simulink library "acc"  (R2021b)
settings: Solver=VariableStepAuto  StartTime=0.0  StopTime=10.0  RelTol=1e-3
undefined symbols (not defined in the file or in its folder): AACC_EHPSSpdCtrlMode_X_enum, AACC_EHPSSpdCtrlMode_Y_rad, ENUM__SASCALED_CALED, ENUM_BRAKEPEDAL_RELEASED, ENUM_CACENABLESTS_RUN, ENUM_DCDCENABLESTS_RUN, ENUM_EHPSCTRLMODE_FULLPWR, ENUM_EHPSCTRLMODE_NORMAL, ENUM_EHPSCTRLMODE_STEP1, ENUM_EHPSCTRLMODE_ZERO, ENUM_EHPSENABLESTS_INITIAL, ENUM_EHPSENABLESTS_READY, ENUM_EHPSENABLESTS_RUN, ENUM_PMMMODE_DRIVE, ENUM_PMMMODE_POWERUP, ENUM_TARGETGEAR_NEUTRAL, FALSE, KACC_AirPressInvalid_kpa, KACC_CACEnableFailTime_s, KACC_CACOverrunRcvTime_s, KACC_CACOverrunTime_min, KACC_CACOverTempDelayTime_s, KACC_CACOverTempRcv_s, KACC_CACPresLow_kPa, KACC_CACPressureSWRev_flg, KACC_CACPresWarn_kPa, KACC_CACPresWarn_ovrdflg_flg, KACC_CACPresWarn_ovrdval_flg, KACC_CACStopTime_s, KACC_CACTemp_C, KACC_CACTempRev_C, KACC_CACTempStop_C, KACC_CACTempWarn_C, KACC_CACValid_flg, KACC_CP2VAutoTracH_enum, KACC_CP2VDamStiffReqFA_pct, KACC_CP2VDamStiffReqLA_pct, KACC_CP2VDamStiffReqRA_pct, KACC_CP2VKneeCtrlMReq_enum, KACC_CP2VKneeReqFA_enum, KACC_CP2VKneeReqRA_enum, KACC_CP2VKneeReqRSide_enum, KACC_CP2VLA1PosCmd_enum, KACC_CP2VLA2PosCmd_enum, KACC_CP2VLvCtrlModeReq_enum, KACC_CP2VNLvReqFA_enum, KACC_CP2VNLvReqRA_enum, KACC_DCDCErrLvHoldtime_s, KACC_DTCACCReset_flg, KACC_DTCCACOverrun_cnt, KACC_EACErrLvHoldtime_s, KACC_ECASKneeSideSW_flg, KACC_EcasSw1Down_flg, KACC_EcasSw1Up_flg, KACC_EcasSw2M2_flg, KACC_EcasSw2Stop_flg, KACC_EcasSw3Knee_flg, KACC_EcasSw3M1_flg, KACC_EcasSwDebounceTime_s, KACC_ECASSwitch_flg ... (+30)
libraries: hcu_lib x20, simulink x3
(part 2 of 3)

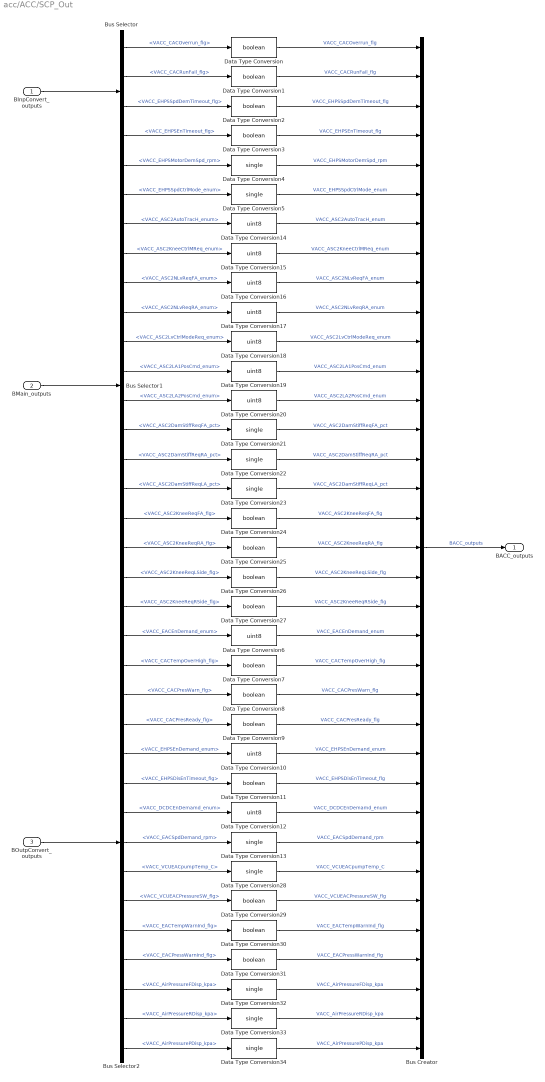
== system acc/ACC/SCP_Out ==
  BInpConvert_outputs : Inport
  BMain_outputs : Inport  Port=2
  BOutpConvert_outputs : Inport  Port=3
  Bus Creator : BusCreator  Inputs=35  OutDataTypeStr=Bus:BACC_outputs  NonVirtualBus=on
  Bus Selector : BusSelector  OutputSignals=VACC_CACOverrun_flg,VACC_CACRunFail_flg,VACC_EHPSSpdDemTimeout_flg,VACC_EHPSEnTimeout_flg
  Bus Selector1 : BusSelector  OutputSignals=VACC_EHPSMotorDemSpd_rpm,VACC_EHPSSpdCtrlMode_enum,VACC_ASC2AutoTracH_enum,VACC_ASC2KneeCtrlMReq_enum,VACC_ASC2NLvReqFA_enum,VACC_ASC2NLvReqRA_enum,VACC_ASC2LvCtrlModeReq_enum,VACC_ASC2LA1PosCmd_enum,VACC_ASC2LA2PosCmd_enum,VACC_ASC2DamStiffReqFA_pct,VACC_ASC2DamStiffReqRA_pct,VACC_ASC2DamStiffReqLA_pct,VACC_ASC2KneeReqFA_flg,VACC_ASC2KneeReqRA_flg,VACC_ASC2KneeReqLSide_flg,VACC_ASC2KneeReqRSide_flg
  Bus Selector2 : BusSelector  OutputSignals=VACC_EACEnDemand_enum,VACC_CACTempOverHigh_flg,VACC_CACPresWarn_flg,VACC_CACPresReady_flg,VACC_EHPSEnDemand_enum,VACC_EHPSDisEnTimeout_flg,VACC_DCDCEnDemamd_enum,VACC_EACSpdDemand_rpm,VACC_VCUEACpumpTemp_C,VACC_VCUEACPressureSW_flg,VACC_EACTempWarnInd_flg,VACC_EACPressWarnInd_flg,VACC_AirPressureFDisp_kpa,VACC_AirPressureRDisp_kpa,VACC_AirPressurePDisp_kpa
  Data Type Conversion{,1..3,7..9,11,24..27,29..31} (15 alike) : DataTypeConversion  OutDataTypeStr=boolean
  Data Type Conversion{6,10,12,14..20} (10 alike) : DataTypeConversion  OutDataTypeStr=uint8
  Data Type Conversion{4..5,13,21..23,28,32..34} (10 alike) : DataTypeConversion  OutDataTypeStr=single
  BACC_outputs : Outport
  wires:
  BInpConvert_outputs/1 -> Bus Selector/1
  BMain_outputs/1 -> Bus Selector1/1
  BOutpConvert_outputs/1 -> Bus Selector2/1
  Bus Selector/1 -> Data Type Conversion/1  "<VACC_CACOverrun_flg>"
  Bus Selector/2 -> Data Type Conversion1/1  "<VACC_CACRunFail_flg>"
  Bus Selector/3 -> Data Type Conversion2/1  "<VACC_EHPSSpdDemTimeout_flg>"
  Bus Selector/4 -> Data Type Conversion3/1  "<VACC_EHPSEnTimeout_flg>"
  Bus Selector1/1 -> Data Type Conversion4/1  "<VACC_EHPSMotorDemSpd_rpm>"
  Bus Selector1/2 -> Data Type Conversion5/1  "<VACC_EHPSSpdCtrlMode_enum>"
  Bus Selector2/1 -> Data Type Conversion6/1  "<VACC_EACEnDemand_enum>"
  Bus Selector2/2 -> Data Type Conversion7/1  "<VACC_CACTempOverHigh_flg>"
  Bus Selector2/3 -> Data Type Conversion8/1  "<VACC_CACPresWarn_flg>"
  Bus Selector2/4 -> Data Type Conversion9/1  "<VACC_CACPresReady_flg>"
  Bus Selector2/5 -> Data Type Conversion10/1  "<VACC_EHPSEnDemand_enum>"
  Bus Selector2/6 -> Data Type Conversion11/1  "<VACC_EHPSDisEnTimeout_flg>"
  Bus Selector2/7 -> Data Type Conversion12/1  "<VACC_DCDCEnDemamd_enum>"
  Bus Selector2/8 -> Data Type Conversion13/1  "<VACC_EACSpdDemand_rpm>"
  Data Type Conversion/1 -> Bus Creator/1  "VACC_CACOverrun_flg"
  Data Type Conversion1/1 -> Bus Creator/2  "VACC_CACRunFail_flg"
  Data Type Conversion2/1 -> Bus Creator/3  "VACC_EHPSSpdDemTimeout_flg"
  Data Type Conversion3/1 -> Bus Creator/4  "VACC_EHPSEnTimeout_flg"
  Data Type Conversion4/1 -> Bus Creator/5  "VACC_EHPSMotorDemSpd_rpm"
  Data Type Conversion5/1 -> Bus Creator/6  "VACC_EHPSSpdCtrlMode_enum"
  Bus Creator/1 -> BACC_outputs/1  "BACC_outputs"
  Bus Selector1/3 -> Data Type Conversion14/1  "<VACC_ASC2AutoTracH_enum>"
  Bus Selector1/4 -> Data Type Conversion15/1  "<VACC_ASC2KneeCtrlMReq_enum>"
  Bus Selector1/5 -> Data Type Conversion16/1  "<VACC_ASC2NLvReqFA_enum>"
  Bus Selector1/6 -> Data Type Conversion17/1  "<VACC_ASC2NLvReqRA_enum>"
  Bus Selector1/7 -> Data Type Conversion18/1  "<VACC_ASC2LvCtrlModeReq_enum>"
  Bus Selector1/8 -> Data Type Conversion19/1  "<VACC_ASC2LA1PosCmd_enum>"
  Bus Selector1/9 -> Data Type Conversion20/1  "<VACC_ASC2LA2PosCmd_enum>"
  Bus Selector1/10 -> Data Type Conversion21/1  "<VACC_ASC2DamStiffReqFA_pct>"
  Bus Selector1/11 -> Data Type Conversion22/1  "<VACC_ASC2DamStiffReqRA_pct>"
  Bus Selector1/12 -> Data Type Conversion23/1  "<VACC_ASC2DamStiffReqLA_pct>"
  Bus Selector1/13 -> Data Type Conversion24/1  "<VACC_ASC2KneeReqFA_flg>"
  Bus Selector1/14 -> Data Type Conversion25/1  "<VACC_ASC2KneeReqRA_flg>"
  Bus Selector1/15 -> Data Type Conversion26/1  "<VACC_ASC2KneeReqLSide_flg>"
  Bus Selector1/16 -> Data Type Conversion27/1  "<VACC_ASC2KneeReqRSide_flg>"
  Bus Selector2/9 -> Data Type Conversion28/1  "<VACC_VCUEACpumpTemp_C>"
  Bus Selector2/10 -> Data Type Conversion29/1  "<VACC_VCUEACPressureSW_flg>"
  Bus Selector2/11 -> Data Type Conversion30/1  "<VACC_EACTempWarnInd_flg>"
  Bus Selector2/12 -> Data Type Conversion31/1  "<VACC_EACPressWarnInd_flg>"
  Bus Selector2/13 -> Data Type Conversion32/1  "<VACC_AirPressureFDisp_kpa>"
  Bus Selector2/14 -> Data Type Conversion33/1  "<VACC_AirPressureRDisp_kpa>"
  Bus Selector2/15 -> Data Type Conversion34/1  "<VACC_AirPressurePDisp_kpa>"
  Data Type Conversion14/1 -> Bus Creator/7  "VACC_ASC2AutoTracH_enum"
  Data Type Conversion15/1 -> Bus Creator/8  "VACC_ASC2KneeCtrlMReq_enum"
  Data Type Conversion16/1 -> Bus Creator/9  "VACC_ASC2NLvReqFA_enum"
  Data Type Conversion17/1 -> Bus Creator/10  "VACC_ASC2NLvReqRA_enum"
  Data Type Conversion18/1 -> Bus Creator/11  "VACC_ASC2LvCtrlModeReq_enum"
  Data Type Conversion19/1 -> Bus Creator/12  "VACC_ASC2LA1PosCmd_enum"
  Data Type Conversion20/1 -> Bus Creator/13  "VACC_ASC2LA2PosCmd_enum"
  Data Type Conversion21/1 -> Bus Creator/14  "VACC_ASC2DamStiffReqFA_pct"
  Data Type Conversion22/1 -> Bus Creator/15  "VACC_ASC2DamStiffReqRA_pct"
  Data Type Conversion23/1 -> Bus Creator/16  "VACC_ASC2DamStiffReqLA_pct"
  Data Type Conversion24/1 -> Bus Creator/17  "VACC_ASC2KneeReqFA_flg"
  Data Type Conversion25/1 -> Bus Creator/18  "VACC_ASC2KneeReqRA_flg"
  Data Type Conversion26/1 -> Bus Creator/19  "VACC_ASC2KneeReqLSide_flg"
  Data Type Conversion27/1 -> Bus Creator/20  "VACC_ASC2KneeReqRSide_flg"
  Data Type Conversion6/1 -> Bus Creator/21  "VACC_EACEnDemand_enum"
  Data Type Conversion7/1 -> Bus Creator/22  "VACC_CACTempOverHigh_flg"
  Data Type Conversion8/1 -> Bus Creator/23  "VACC_CACPresWarn_flg"
  Data Type Conversion9/1 -> Bus Creator/24  "VACC_CACPresReady_flg"
  Data Type Conversion10/1 -> Bus Creator/25  "VACC_EHPSEnDemand_enum"
  Data Type Conversion11/1 -> Bus Creator/26  "VACC_EHPSDisEnTimeout_flg"
  Data Type Conversion12/1 -> Bus Creator/27  "VACC_DCDCEnDemamd_enum"
  Data Type Conversion13/1 -> Bus Creator/28  "VACC_EACSpdDemand_rpm"
  Data Type Conversion28/1 -> Bus Creator/29  "VACC_VCUEACpumpTemp_C"
  Data Type Conversion29/1 -> Bus Creator/30  "VACC_VCUEACPressureSW_flg"
  Data Type Conversion30/1 -> Bus Creator/31  "VACC_EACTempWarnInd_flg"
  Data Type Conversion31/1 -> Bus Creator/32  "VACC_EACPressWarnInd_flg"
  Data Type Conversion32/1 -> Bus Creator/33  "VACC_AirPressureFDisp_kpa"
  Data Type Conversion33/1 -> Bus Creator/34  "VACC_AirPressureRDisp_kpa"
  Data Type Conversion34/1 -> Bus Creator/35  "VACC_AirPressurePDisp_kpa"

== system acc/ACC/Input_Convert/ EcasSw1Down Debounce ==
  signal_raw : Inport
  time_limit : Inport  Port=2
  time_step : Inport  Port=3
  Add : Sum
  Add1 : Sum
  Constant : Constant  Value=FALSE
  Constant1 : Constant  Value=0
  Relational Operator : RelationalOperator  OutDataTypeStr=boolean  RndMeth=Simplest
  Switch : Switch  Criteria=u2 ~= 0
      settings: AttributesFormatString=%<Criteria>
  Switch1 : Switch  Criteria=u2 ~= 0
      settings: AttributesFormatString=%<Criteria>
  Unit Delay : UnitDelay  SampleTime=-1  HasFrameUpgradeWarning=on
  signal_out : Outport
  wires:
  signal_raw/1 -> Switch1/2, Switch/2
  Constant/1 -> Switch/3
  time_step/1 -> Add1/2, Add/1
  Unit Delay/1 -> Add/2
  Relational Operator/1 -> Switch/1
  Switch1/1 -> Unit Delay/1, Relational Operator/1
  Add/1 -> Switch1/1
  Constant1/1 -> Switch1/3
  Switch/1 -> signal_out/1
  time_limit/1 -> Add1/1
  Add1/1 -> Relational Operator/2

== system acc/ACC/Input_Convert/ EcasSw1Up Debounce ==
  signal_raw : Inport
  time_limit : Inport  Port=2
  time_step : Inport  Port=3
  Add : Sum
  Add1 : Sum
  Constant : Constant  Value=FALSE
  Constant1 : Constant  Value=0
  Relational Operator : RelationalOperator  OutDataTypeStr=boolean  RndMeth=Simplest
  Switch : Switch  Criteria=u2 ~= 0
      settings: AttributesFormatString=%<Criteria>
  Switch1 : Switch  Criteria=u2 ~= 0
      settings: AttributesFormatString=%<Criteria>
  Unit Delay : UnitDelay  SampleTime=-1  HasFrameUpgradeWarning=on
  signal_out : Outport
  wires:
  signal_raw/1 -> Switch1/2, Switch/2
  Constant/1 -> Switch/3
  time_step/1 -> Add1/2, Add/1
  Unit Delay/1 -> Add/2
  Relational Operator/1 -> Switch/1
  Switch1/1 -> Unit Delay/1, Relational Operator/1
  Add/1 -> Switch1/1
  Constant1/1 -> Switch1/3
  Switch/1 -> signal_out/1
  time_limit/1 -> Add1/1
  Add1/1 -> Relational Operator/2

== system acc/ACC/Input_Convert/ EcasSw2Stop Debounce ==
  signal_raw : Inport
  time_limit : Inport  Port=2
  time_step : Inport  Port=3
  Add : Sum
  Add1 : Sum
  Constant : Constant  Value=FALSE
  Constant1 : Constant  Value=0
  Relational Operator : RelationalOperator  OutDataTypeStr=boolean  RndMeth=Simplest
  Switch : Switch  Criteria=u2 ~= 0
      settings: AttributesFormatString=%<Criteria>
  Switch1 : Switch  Criteria=u2 ~= 0
      settings: AttributesFormatString=%<Criteria>
  Unit Delay : UnitDelay  SampleTime=-1  HasFrameUpgradeWarning=on
  signal_out : Outport
  wires:
  signal_raw/1 -> Switch1/2, Switch/2
  Constant/1 -> Switch/3
  time_step/1 -> Add1/2, Add/1
  Unit Delay/1 -> Add/2
  Relational Operator/1 -> Switch/1
  Switch1/1 -> Unit Delay/1, Relational Operator/1
  Add/1 -> Switch1/1
  Constant1/1 -> Switch1/3
  Switch/1 -> signal_out/1
  time_limit/1 -> Add1/1
  Add1/1 -> Relational Operator/2

== system acc/ACC/Input_Convert/EcasSw2M2 Debounce ==
  signal_raw : Inport
  time_limit : Inport  Port=2
  time_step : Inport  Port=3
  Add : Sum
  Add1 : Sum
  Constant : Constant  Value=FALSE
  Constant1 : Constant  Value=0
  Relational Operator : RelationalOperator  OutDataTypeStr=boolean  RndMeth=Simplest
  Switch : Switch  Criteria=u2 ~= 0
      settings: AttributesFormatString=%<Criteria>
  Switch1 : Switch  Criteria=u2 ~= 0
      settings: AttributesFormatString=%<Criteria>
  Unit Delay : UnitDelay  SampleTime=-1  HasFrameUpgradeWarning=on
  signal_out : Outport
  wires:
  signal_raw/1 -> Switch1/2, Switch/2
  Constant/1 -> Switch/3
  time_step/1 -> Add1/2, Add/1
  Unit Delay/1 -> Add/2
  Relational Operator/1 -> Switch/1
  Switch1/1 -> Unit Delay/1, Relational Operator/1
  Add/1 -> Switch1/1
  Constant1/1 -> Switch1/3
  Switch/1 -> signal_out/1
  time_limit/1 -> Add1/1
  Add1/1 -> Relational Operator/2

== system acc/ACC/Input_Convert/EcasSw3Knee Debounce ==
  signal_raw : Inport
  time_limit : Inport  Port=2
  time_step : Inport  Port=3
  Add : Sum
  Add1 : Sum
  Constant : Constant  Value=FALSE
  Constant1 : Constant  Value=0
  Relational Operator : RelationalOperator  OutDataTypeStr=boolean  RndMeth=Simplest
  Switch : Switch  Criteria=u2 ~= 0
      settings: AttributesFormatString=%<Criteria>
  Switch1 : Switch  Criteria=u2 ~= 0
      settings: AttributesFormatString=%<Criteria>
  Unit Delay : UnitDelay  SampleTime=-1  HasFrameUpgradeWarning=on
  signal_out : Outport
  wires:
  signal_raw/1 -> Switch1/2, Switch/2
  Constant/1 -> Switch/3
  time_step/1 -> Add1/2, Add/1
  Unit Delay/1 -> Add/2
  Relational Operator/1 -> Switch/1
  Switch1/1 -> Unit Delay/1, Relational Operator/1
  Add/1 -> Switch1/1
  Constant1/1 -> Switch1/3
  Switch/1 -> signal_out/1
  time_limit/1 -> Add1/1
  Add1/1 -> Relational Operator/2

== system acc/ACC/Input_Convert/EcasSw3M1 Debounce ==
  signal_raw : Inport
  time_limit : Inport  Port=2
  time_step : Inport  Port=3
  Add : Sum
  Add1 : Sum
  Constant : Constant  Value=FALSE
  Constant1 : Constant  Value=0
  Relational Operator : RelationalOperator  OutDataTypeStr=boolean  RndMeth=Simplest
  Switch : Switch  Criteria=u2 ~= 0
      settings: AttributesFormatString=%<Criteria>
  Switch1 : Switch  Criteria=u2 ~= 0
      settings: AttributesFormatString=%<Criteria>
  Unit Delay : UnitDelay  SampleTime=-1  HasFrameUpgradeWarning=on
  signal_out : Outport
  wires:
  signal_raw/1 -> Switch1/2, Switch/2
  Constant/1 -> Switch/3
  time_step/1 -> Add1/2, Add/1
  Unit Delay/1 -> Add/2
  Relational Operator/1 -> Switch/1
  Switch1/1 -> Unit Delay/1, Relational Operator/1
  Add/1 -> Switch1/1
  Constant1/1 -> Switch1/3
  Switch/1 -> signal_out/1
  time_limit/1 -> Add1/1
  Add1/1 -> Relational Operator/2

== system acc/ACC/Input_Convert/Switch hold ==
  signal_in : Inport
  hold_time : Inport  Port=2
  time_step : Inport  Port=3
  Add : Sum
  Constant1 : Constant  Value=0
  Constant3 : Constant  Value=0
  Constant4 : Constant
  Detect Increase : simulink/Logic and Bit Operations/Detect Increase  vinit=0.0  OutDataTypeStr=boolean
  Relational Operator : RelationalOperator  OutDataTypeStr=boolean  RndMeth=Simplest
  Switch1 : Switch  Criteria=u2 ~= 0
      settings: AttributesFormatString=%<Criteria>
  Switch2 : Switch  Criteria=u2 ~= 0
      settings: AttributesFormatString=%<Criteria>
  Switch3 : Switch  Criteria=u2 ~= 0
      settings: AttributesFormatString=%<Criteria>
  Unit Delay : UnitDelay  SampleTime=-1  HasFrameUpgradeWarning=on
  Unit Delay1 : UnitDelay  SampleTime=-1  HasFrameUpgradeWarning=on
  signal_out : Outport
  wires:
  signal_in/1 -> Detect Increase/1
  Detect Increase/1 -> Switch1/2
  Unit Delay/1 -> Switch1/3
  Switch2/1 -> signal_out/1, Unit Delay/1
  Relational Operator/1 -> Switch2/2
  hold_time/1 -> Relational Operator/2
  Switch1/1 -> Switch3/2, Switch2/3
  Switch3/1 -> Unit Delay1/1, Relational Operator/1
  Unit Delay1/1 -> Add/2
  time_step/1 -> Add/1
  Add/1 -> Switch3/1
  Constant1/1 -> Switch3/3
  Constant3/1 -> Switch2/1
  Constant4/1 -> Switch1/1

== system acc/ACC/Input_Convert/Switch hold1 ==
  signal_in : Inport
  hold_time : Inport  Port=2
  time_step : Inport  Port=3
  Add : Sum
  Constant1 : Constant  Value=0
  Constant3 : Constant  Value=0
  Constant4 : Constant
  Detect Increase : simulink/Logic and Bit Operations/Detect Increase  vinit=0.0  OutDataTypeStr=boolean
  Relational Operator : RelationalOperator  OutDataTypeStr=boolean  RndMeth=Simplest
  Switch1 : Switch  Criteria=u2 ~= 0
      settings: AttributesFormatString=%<Criteria>
  Switch2 : Switch  Criteria=u2 ~= 0
      settings: AttributesFormatString=%<Criteria>
  Switch3 : Switch  Criteria=u2 ~= 0
      settings: AttributesFormatString=%<Criteria>
  Unit Delay : UnitDelay  SampleTime=-1  HasFrameUpgradeWarning=on
  Unit Delay1 : UnitDelay  SampleTime=-1  HasFrameUpgradeWarning=on
  signal_out : Outport
  wires:
  signal_in/1 -> Detect Increase/1
  Detect Increase/1 -> Switch1/2
  Unit Delay/1 -> Switch1/3
  Switch2/1 -> signal_out/1, Unit Delay/1
  Relational Operator/1 -> Switch2/2
  hold_time/1 -> Relational Operator/2
  Switch1/1 -> Switch3/2, Switch2/3
  Switch3/1 -> Unit Delay1/1, Relational Operator/1
  Unit Delay1/1 -> Add/2
  time_step/1 -> Add/1
  Add/1 -> Switch3/1
  Constant1/1 -> Switch3/3
  Constant3/1 -> Switch2/1
  Constant4/1 -> Switch1/1

== system acc/ACC/Input_Convert/Switch hold3 ==
  signal_in : Inport
  hold_time : Inport  Port=2
  time_step : Inport  Port=3
  Add : Sum
  Constant1 : Constant  Value=0
  Constant3 : Constant  Value=0
  Constant4 : Constant
  Detect Increase : simulink/Logic and Bit Operations/Detect Increase  vinit=0.0  OutDataTypeStr=boolean
  Relational Operator : RelationalOperator  OutDataTypeStr=boolean  RndMeth=Simplest
  Switch1 : Switch  Criteria=u2 ~= 0
      settings: AttributesFormatString=%<Criteria>
  Switch2 : Switch  Criteria=u2 ~= 0
      settings: AttributesFormatString=%<Criteria>
  Switch3 : Switch  Criteria=u2 ~= 0
      settings: AttributesFormatString=%<Criteria>
  Unit Delay : UnitDelay  SampleTime=-1  HasFrameUpgradeWarning=on
  Unit Delay1 : UnitDelay  SampleTime=-1  HasFrameUpgradeWarning=on
  signal_out : Outport
  wires:
  signal_in/1 -> Detect Increase/1
  Detect Increase/1 -> Switch1/2
  Unit Delay/1 -> Switch1/3
  Switch2/1 -> signal_out/1, Unit Delay/1
  Relational Operator/1 -> Switch2/2
  hold_time/1 -> Relational Operator/2
  Switch1/1 -> Switch3/2, Switch2/3
  Switch3/1 -> Unit Delay1/1, Relational Operator/1
  Unit Delay1/1 -> Add/2
  time_step/1 -> Add/1
  Add/1 -> Switch3/1
  Constant1/1 -> Switch3/3
  Constant3/1 -> Switch2/1
  Constant4/1 -> Switch1/1

== system acc/ACC/Input_Convert/Trigger ==
  task_time_s : Inport
  DectectTime : Inport  Port=2
  Add1 : Sum
  Constant62 : Constant  Value=ZERO_FLOAT
  NOT : Logic  Operator=NOT  AllPortsSameDT=off  OutDataTypeStr=boolean
  Relational Operator2 : RelationalOperator  OutDataTypeStr=boolean  RndMeth=Simplest
  Switch6 : Switch  Criteria=u2 ~= 0
      settings: AttributesFormatString=%<Criteria>
  Unit Delay1 : UnitDelay  InitialCondition=boolean(0)  SampleTime=-1  HasFrameUpgradeWarning=on
      settings: AttributesFormatString=%<InitialCondition>
  Unit Delay2 : UnitDelay  InitialCondition=single(0)  SampleTime=-1  HasFrameUpgradeWarning=on
      settings: AttributesFormatString=%<InitialCondition>
  ActionFlag : Outport
  wires:
  NOT/1 -> Switch6/2
  Unit Delay1/1 -> NOT/1
  Switch6/1 -> Relational Operator2/1, Unit Delay2/1
  task_time_s/1 -> Add1/2
  DectectTime/1 -> Relational Operator2/2
  Unit Delay2/1 -> Add1/1
  Add1/1 -> Switch6/1
  Constant62/1 -> Switch6/3
  Relational Operator2/1 -> ActionFlag/1, Unit Delay1/1

== system acc/ACC/Main/DCDC Control ==
  BSCP_In_outputs : Inport
  BInpConvert_outputs : Inport  Port=2
  AND : Logic  AllPortsSameDT=off  OutDataTypeStr=boolean
  Bus Selector : BusSelector  OutputSignals=VPMM_SysPowerMode_enum,task_time_s,VINP_DCDCEnSta_enum,VDMM_DTCDCDCErrLv_flg,VDMM_DTCDCDCRlyNoFB_flg,VPMM_PMMDCDCEnableDem_flg
  Constant : Constant  Value=FALSE
  Constant1 : Constant  Value=ENUM_DCDCENABLESTS_RUN
  Constant2 : Constant  Value=ENUM_PMMMODE_DRIVE
  Constant7 : Constant  Value=KACC_DCDCErrLvHoldtime_s
  Equal : RelationalOperator  Operator=~=  OutDataTypeStr=boolean  RndMeth=Simplest
  Equal1 : RelationalOperator  Operator===  OutDataTypeStr=boolean  RndMeth=Simplest
  OR : Logic  Operator=OR  AllPortsSameDT=off  OutDataTypeStr=boolean
  Recover : hcu_lib/Basic_Blocks/Recover  SystemSampleTime=-1  VariantActivationTime=update diagram  Latency=0  AutoFrameSizeCalculation=off
      settings: SourceProductName=HCU Relative Block Library
  SR_Latch : hcu_lib/Basic_Blocks/SR_Latch
      settings: SourceProductName=HCU Relative Block Library
  Switch : Switch  Criteria=u2 ~= 0
      settings: AttributesFormatString=%<Criteria>
  Terminator : Terminator
  VACC_DCDCEnableDem_flg : Outport
  wires:
  BSCP_In_outputs/1 -> Bus Selector/1
  BInpConvert_outputs/1 -> Terminator/1
  Recover/1 -> SR_Latch/2
  Constant/1 -> Switch/1
  Equal/1 -> Recover/2
  Constant7/1 -> Recover/3
  SR_Latch/1 -> OR/1
  OR/1 -> Switch/2
  AND/1 -> OR/2
  Constant1/1 -> Equal/2
  Constant2/1 -> Equal1/1
  Equal1/1 -> AND/1
  [VDMM_DTCDCDCErrLv_flg] -> SR_Latch/1
  [task_time_s] -> Recover/1
  [VINP_DCDCEnSta_enum] -> Equal/1
  [VPMM_SysPowerMode_enum] -> Equal1/2
  [VDMM_DTCDCDCRlyNoFB_flg] -> AND/2
  [VPMM_PMMDCDCEnableDem_flg] -> Switch/3
  Bus Selector/1 -> [VPMM_SysPowerMode_enum]  "<VPMM_SysPowerMode_enum>"
  Bus Selector/2 -> [task_time_s]  "<task_time_s>"
  Bus Selector/3 -> [VINP_DCDCEnSta_enum]  "<VINP_DCDCEnSta_enum>"
  Bus Selector/4 -> [VDMM_DTCDCDCErrLv_flg]  "<VDMM_DTCDCDCErrLv_flg>"
  Bus Selector/5 -> [VDMM_DTCDCDCRlyNoFB_flg]  "<VDMM_DTCDCDCRlyNoFB_flg>"
  Bus Selector/6 -> [VPMM_PMMDCDCEnableDem_flg]  "<VPMM_PMMDCDCEnableDem_flg>"
  Switch/1 -> [VACC_DCDCEnableDem_flg]  "VACC_DCDCEnableDem_flg"
  [VACC_DCDCEnableDem_flg] -> VACC_DCDCEnableDem_flg/1

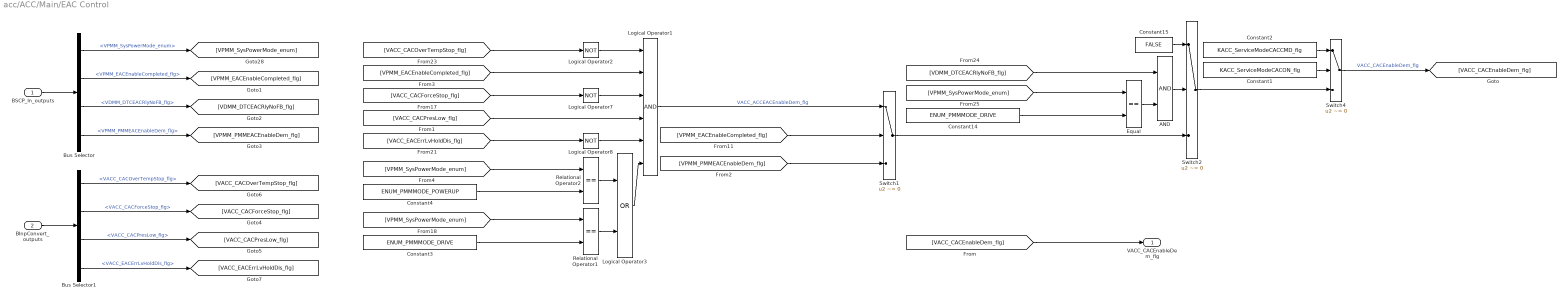
== system acc/ACC/Main/EAC Control ==
  BSCP_In_outputs : Inport
  BInpConvert_outputs : Inport  Port=2
  AND : Logic  AllPortsSameDT=off  OutDataTypeStr=boolean
  Bus Selector : BusSelector  OutputSignals=VPMM_SysPowerMode_enum,VPMM_EACEnableCompleted_flg,VDMM_DTCEACRlyNoFB_flg,VPMM_PMMEACEnableDem_flg
  Bus Selector1 : BusSelector  OutputSignals=VACC_CACOverTempStop_flg,VACC_CACForceStop_flg,VACC_CACPresLow_flg,VACC_EACErrLvHoldDis_flg
  Constant1 : Constant  Value=KACC_ServiceModeCACON_flg  SampleTime=-1
  Constant14 : Constant  Value=ENUM_PMMMODE_DRIVE  SampleTime=-1
  Constant15 : Constant  Value=FALSE
  Constant2 : Constant  Value=KACC_ServiceModeCACCMD_flg  SampleTime=-1
  Constant3 : Constant  Value=ENUM_PMMMODE_DRIVE  SampleTime=-1
  Constant4 : Constant  Value=ENUM_PMMMODE_POWERUP  SampleTime=-1
  Equal : RelationalOperator  Operator===  OutDataTypeStr=boolean  RndMeth=Simplest
  Logical Operator1 : Logic  Inputs=6  AllPortsSameDT=off  OutDataTypeStr=boolean
  Logical Operator2 : Logic  Operator=NOT  AllPortsSameDT=off  OutDataTypeStr=boolean
  Logical Operator3 : Logic  Operator=OR  AllPortsSameDT=off  OutDataTypeStr=boolean
  Logical Operator7 : Logic  Operator=NOT  AllPortsSameDT=off  OutDataTypeStr=boolean
  Logical Operator8 : Logic  Operator=NOT  AllPortsSameDT=off  OutDataTypeStr=boolean
  Relational Operator1 : RelationalOperator  Operator===  OutDataTypeStr=boolean  RndMeth=Nearest
  Relational Operator2 : RelationalOperator  Operator===  OutDataTypeStr=boolean  RndMeth=Nearest
  Switch1 : Switch  Criteria=u2 ~= 0
      settings: AttributesFormatString=%<Criteria>
  Switch2 : Switch  Criteria=u2 ~= 0
      settings: AttributesFormatString=%<Criteria>
  Switch4 : Switch  Criteria=u2 ~= 0
      settings: AttributesFormatString=%<Criteria>
  VACC_CACEnableDem_flg : Outport
  wires:
  Relational Operator1/1 -> Logical Operator3/2
  Logical Operator8/1 -> Logical Operator1/5
  [VPMM_SysPowerMode_enum] -> Relational Operator2/1
  Logical Operator7/1 -> Logical Operator1/3
  [VACC_CACPresLow_flg] -> Logical Operator1/4
  Switch2/1 -> Switch4/3
  [VACC_EACErrLvHoldDis_flg] -> Logical Operator8/1
  [VACC_CACOverTempStop_flg] -> Logical Operator2/1
  [VPMM_EACEnableCompleted_flg] -> Logical Operator1/2
  Logical Operator2/1 -> Logical Operator1/1
  [VPMM_SysPowerMode_enum] -> Relational Operator1/1
  [VACC_CACForceStop_flg] -> Logical Operator7/1
  Switch1/1 -> Switch2/3
  Constant4/1 -> Relational Operator2/2
  Logical Operator1/1 -> Switch1/1  "VACC_ACCEACEnableDem_flg"
  Relational Operator2/1 -> Logical Operator3/1
  Logical Operator3/1 -> Logical Operator1/6
  Constant3/1 -> Relational Operator1/2
  Equal/1 -> AND/2
  [VPMM_SysPowerMode_enum] -> Equal/1
  Constant15/1 -> Switch2/1
  AND/1 -> Switch2/2
  [VPMM_EACEnableCompleted_flg] -> Switch1/2
  Constant1/1 -> Switch4/2
  Constant14/1 -> Equal/2
  [VDMM_DTCEACRlyNoFB_flg] -> AND/1
  BSCP_In_outputs/1 -> Bus Selector/1
  [VPMM_PMMEACEnableDem_flg] -> Switch1/3
  Bus Selector/1 -> [VPMM_SysPowerMode_enum]  "<VPMM_SysPowerMode_enum>"
  Bus Selector/2 -> [VPMM_EACEnableCompleted_flg]  "<VPMM_EACEnableCompleted_flg>"
  Bus Selector/3 -> [VDMM_DTCEACRlyNoFB_flg]  "<VDMM_DTCEACRlyNoFB_flg>"
  Bus Selector/4 -> [VPMM_PMMEACEnableDem_flg]  "<VPMM_PMMEACEnableDem_flg>"
  BInpConvert_outputs/1 -> Bus Selector1/1
  Bus Selector1/2 -> [VACC_CACForceStop_flg]  "<VACC_CACForceStop_flg>"
  Bus Selector1/3 -> [VACC_CACPresLow_flg]  "<VACC_CACPresLow_flg>"
  Bus Selector1/1 -> [VACC_CACOverTempStop_flg]  "<VACC_CACOverTempStop_flg>"
  Bus Selector1/4 -> [VACC_EACErrLvHoldDis_flg]  "<VACC_EACErrLvHoldDis_flg>"
  Constant2/1 -> Switch4/1
  Switch4/1 -> [VACC_CACEnableDem_flg]  "VACC_CACEnableDem_flg"
  [VACC_CACEnableDem_flg] -> VACC_CACEnableDem_flg/1

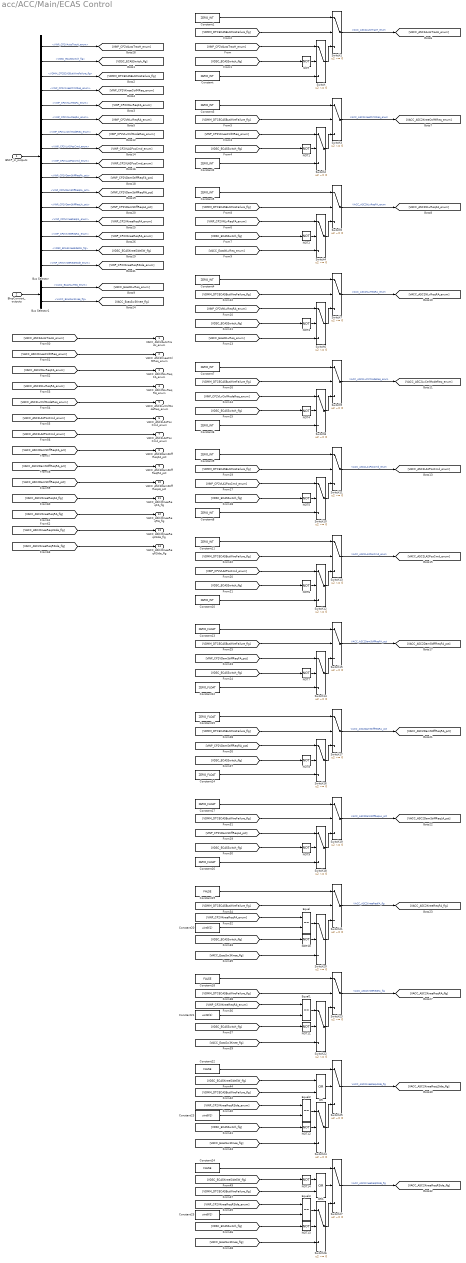
== system acc/ACC/Main/ECAS Control ==
  BSCP_In_outputs : Inport
  BInpConvert_outputs : Inport  Port=2
  Bus Selector : BusSelector  OutputSignals=VINP_CP2VAutoTracH_enum,VDSC_ECASSwitch_flg,VDMM_DTCECASButWireFailure_flg,VINP_CP2VKneeCtrlMReq_enum,VINP_CP2VNLvReqFA_enum,VINP_CP2VNLvReqRA_enum,VINP_CP2VLvCtrlModeReq_enum,VINP_CP2VLA1PosCmd_enum,VINP_CP2VLA2PosCmd_enum,VINP_CP2VDamStiffReqFA_pct,VINP_CP2VDamStiffReqRA_pct,VINP_CP2VDamStiffReqLA_pct,VINP_CP2VKneeReqFA_enum,VINP_CP2VKneeReqRA_enum,VDSC_ECASKneeSideSW_flg,VINP_CP2VKneeReqRSide_enum
  Bus Selector1 : BusSelector  OutputSignals=VACC_EcasNLvReq_enum,VACC_EcasSw3Knee_flg
  Constant{,1..11} (12 alike) : Constant  Value=ZERO_INT
  Constant{12..17} (6 alike) : Constant  Value=ZERO_FLOAT
  Constant{18..19,22,24} (4 alike) : Constant  Value=FALSE
  Constant{20..21,23,25} (4 alike) : Constant  Value=uint8(1)
  Equal{,1..3} (4 alike) : RelationalOperator  Operator===  OutDataTypeStr=boolean  RndMeth=Simplest
  NOT{,1..14} (15 alike) : Logic  Operator=NOT  AllPortsSameDT=off  OutDataTypeStr=boolean
  OR : Logic  Operator=OR  AllPortsSameDT=off  OutDataTypeStr=boolean
  OR1 : Logic  Operator=OR  AllPortsSameDT=off  OutDataTypeStr=boolean
  Switch{,1..27} (28 alike) : Switch  Criteria=u2 ~= 0
      settings: AttributesFormatString=%<Criteria>
  VACC_ASC2AutoTracH_enum : Outport
  VACC_ASC2KneeCtrlMReq_enum : Outport  Port=2
  VACC_ASC2NLvReqFA_enum : Outport  Port=3
  VACC_ASC2NLvReqRA_enum : Outport  Port=4
  VACC_ASC2LvCtrlModeReq_enum : Outport  Port=5
  VACC_ASC2LA1PosCmd_enum : Outport  Port=6
  VACC_ASC2LA2PosCmd_enum : Outport  Port=7
  VACC_ASC2DamStiffReqFA_pct : Outport  Port=8
  VACC_ASC2DamStiffReqRA_pct : Outport  Port=9
  VACC_ASC2DamStiffReqLA_pct : Outport  Port=10
  VACC_ASC2KneeReqFA_flg : Outport  Port=11
  VACC_ASC2KneeReqRA_flg : Outport  Port=12
  VACC_ASC2KneeReqLSide_flg : Outport  Port=13
  VACC_ASC2KneeReqRSide_flg : Outport  Port=14
  wires:
  Bus Selector/2 -> [VDSC_ECASSwitch_flg]  "<VDSC_ECASSwitch_flg>"
  Bus Selector/1 -> [VINP_CP2VAutoTracH_enum]  "<VINP_CP2VAutoTracH_enum>"
  BSCP_In_outputs/1 -> Bus Selector/1
  [VINP_CP2VAutoTracH_enum] -> Switch/1
  Constant/1 -> Switch/3
  Bus Selector/3 -> [VDMM_DTCECASButWireFailure_flg]  "<VDMM_DTCECASButWireFailure_flg>"
  [VDSC_ECASSwitch_flg] -> NOT/1
  NOT/1 -> Switch/2
  Switch/1 -> Switch1/3
  [VDMM_DTCECASButWireFailure_flg] -> Switch1/2
  Constant1/1 -> Switch1/1
  Switch1/1 -> [VACC_ASC2AutoTracH_enum]  "VACC_ASC2AutoTracH_enum"
  Switch3/1 -> [VACC_ASC2KneeCtrlMReq_enum]  "VACC_ASC2KneeCtrlMReq_enum"
  Constant3/1 -> Switch3/1
  [VDMM_DTCECASButWireFailure_flg] -> Switch3/2
  Switch2/1 -> Switch3/3
  NOT1/1 -> Switch2/2
  [VDSC_ECASSwitch_flg] -> NOT1/1
  Constant2/1 -> Switch2/3
  [VINP_CP2VKneeCtrlMReq_enum] -> Switch2/1
  Bus Selector/4 -> [VINP_CP2VKneeCtrlMReq_enum]  "<VINP_CP2VKneeCtrlMReq_enum>"
  [VINP_CP2VNLvReqFA_enum] -> Switch4/1
  [VDSC_ECASSwitch_flg] -> NOT2/1
  NOT2/1 -> Switch4/2
  Switch4/1 -> Switch5/3
  [VDMM_DTCECASButWireFailure_flg] -> Switch5/2
  Constant5/1 -> Switch5/1
  Switch5/1 -> [VACC_ASC2NLvReqFA_enum]  "VACC_ASC2NLvReqFA_enum"
  Bus Selector/5 -> [VINP_CP2VNLvReqFA_enum]  "<VINP_CP2VNLvReqFA_enum>"
  BInpConvert_outputs/1 -> Bus Selector1/1
  Bus Selector1/1 -> [VACC_EcasNLvReq_enum]  "<VACC_EcasNLvReq_enum>"
  [VACC_EcasNLvReq_enum] -> Switch4/3
  [VACC_EcasNLvReq_enum] -> Switch6/3
  Switch7/1 -> [VACC_ASC2NLvReqRA_enum]  "VACC_ASC2NLvReqRA_enum"
  Constant4/1 -> Switch7/1
  [VDMM_DTCECASButWireFailure_flg] -> Switch7/2
  Switch6/1 -> Switch7/3
  NOT3/1 -> Switch6/2
  [VDSC_ECASSwitch_flg] -> NOT3/1
  [VINP_CP2VNLvReqRA_enum] -> Switch6/1
  Bus Selector/6 -> [VINP_CP2VNLvReqRA_enum]  "<VINP_CP2VNLvReqRA_enum>"
  Switch8/1 -> Switch9/3
  Constant6/1 -> Switch8/3
  [VDMM_DTCECASButWireFailure_flg] -> Switch9/2
  [VDSC_ECASSwitch_flg] -> NOT4/1
  NOT4/1 -> Switch8/2
  [VINP_CP2VLvCtrlModeReq_enum] -> Switch8/1
  Switch9/1 -> [VACC_ASC2LvCtrlModeReq_enum]  "VACC_ASC2LvCtrlModeReq_enum"
  Constant7/1 -> Switch9/1
  Bus Selector/7 -> [VINP_CP2VLvCtrlModeReq_enum]  "<VINP_CP2VLvCtrlModeReq_enum>"
  [VDSC_ECASSwitch_flg] -> NOT5/1
  [VINP_CP2VLA1PosCmd_enum] -> Switch10/1
  NOT5/1 -> Switch10/2
  Switch11/1 -> [VACC_ASC2LA1PosCmd_enum]  "VACC_ASC2LA1PosCmd_enum"
  Constant8/1 -> Switch10/3
  Switch10/1 -> Switch11/3
  Constant9/1 -> Switch11/1
  [VDMM_DTCECASButWireFailure_flg] -> Switch11/2
  Bus Selector/8 -> [VINP_CP2VLA1PosCmd_enum]  "<VINP_CP2VLA1PosCmd_enum>"
  [VDMM_DTCECASButWireFailure_flg] -> Switch13/2
  Constant11/1 -> Switch13/1
  Switch13/1 -> [VACC_ASC2LA2PosCmd_enum]  "VACC_ASC2LA2PosCmd_enum"
  [VINP_CP2VLA2PosCmd_enum] -> Switch12/1
  NOT6/1 -> Switch12/2
  Constant10/1 -> Switch12/3
  Switch12/1 -> Switch13/3
  [VDSC_ECASSwitch_flg] -> NOT6/1
  Bus Selector/9 -> [VINP_CP2VLA2PosCmd_enum]  "<VINP_CP2VLA2PosCmd_enum>"
  [VDSC_ECASSwitch_flg] -> NOT7/1
  Switch14/1 -> Switch15/3
  Constant12/1 -> Switch14/3
  NOT7/1 -> Switch14/2
  [VINP_CP2VDamStiffReqFA_pct] -> Switch14/1
  Switch15/1 -> [VACC_ASC2DamStiffReqFA_pct]  "VACC_ASC2DamStiffReqFA_pct"
  Constant13/1 -> Switch15/1
  [VDMM_DTCECASButWireFailure_flg] -> Switch15/2
  Bus Selector/10 -> [VINP_CP2VDamStiffReqFA_pct]  "<VINP_CP2VDamStiffReqFA_pct>"
  Bus Selector/11 -> [VINP_CP2VDamStiffReqRA_pct]  "<VINP_CP2VDamStiffReqRA_pct>"
  Bus Selector/12 -> [VINP_CP2VDamStiffReqLA_pct]  "<VINP_CP2VDamStiffReqLA_pct>"
  [VDMM_DTCECASButWireFailure_flg] -> Switch17/2
  Constant15/1 -> Switch17/1
  Switch17/1 -> [VACC_ASC2DamStiffReqRA_pct]  "VACC_ASC2DamStiffReqRA_pct"
  [VINP_CP2VDamStiffReqRA_pct] -> Switch16/1
  NOT8/1 -> Switch16/2
  Constant14/1 -> Switch16/3
  Switch16/1 -> Switch17/3
  [VDSC_ECASSwitch_flg] -> NOT8/1
  NOT9/1 -> Switch18/2
  Switch18/1 -> Switch19/3
  Constant17/1 -> Switch19/1
  [VINP_CP2VDamStiffReqLA_pct] -> Switch18/1
  Constant16/1 -> Switch18/3
  Switch19/1 -> [VACC_ASC2DamStiffReqLA_pct]  "VACC_ASC2DamStiffReqLA_pct"
  [VDSC_ECASSwitch_flg] -> NOT9/1
  [VDMM_DTCECASButWireFailure_flg] -> Switch19/2
  NOT10/1 -> Switch20/2
  [VDMM_DTCECASButWireFailure_flg] -> Switch21/2
  [VDSC_ECASSwitch_flg] -> NOT10/1
  Switch21/1 -> [VACC_ASC2KneeReqFA_flg]  "VACC_ASC2KneeReqFA_flg"
  Constant19/1 -> Switch21/1
  Switch20/1 -> Switch21/3
  Equal/1 -> Switch20/1
  [VINP_CP2VKneeReqFA_enum] -> Equal/1
  Constant20/1 -> Equal/2
  Bus Selector1/2 -> [VACC_EcasSw3Knee_flg]  "<VACC_EcasSw3Knee_flg>"
  [VACC_EcasSw3Knee_flg] -> Switch20/3
  Bus Selector/13 -> [VINP_CP2VKneeReqFA_enum]  "<VINP_CP2VKneeReqFA_enum>"
  Bus Selector/14 -> [VINP_CP2VKneeReqRA_enum]  "<VINP_CP2VKneeReqRA_enum>"
  Equal1/1 -> Switch22/1
  [VINP_CP2VKneeReqRA_enum] -> Equal1/1
  [VDSC_ECASSwitch_flg] -> NOT11/1
  Switch23/1 -> [VACC_ASC2KneeReqRA_flg]  "VACC_ASC2KneeReqRA_flg"
  [VDMM_DTCECASButWireFailure_flg] -> Switch23/2
  Constant18/1 -> Switch23/1
  Switch22/1 -> Switch23/3
  NOT11/1 -> Switch22/2
  [VACC_EcasSw3Knee_flg] -> Switch22/3
  Constant21/1 -> Equal1/2
  Bus Selector/15 -> [VDSC_ECASKneeSideSW_flg]  "<VDSC_ECASKneeSideSW_flg>"
  Constant23/1 -> Equal2/2
  NOT12/1 -> Switch24/2
  Switch24/1 -> Switch25/3
  [VDSC_ECASSwitch_flg] -> NOT12/1
  Switch25/1 -> [VACC_ASC2KneeReqLSide_flg]  "VACC_ASC2KneeReqLSide_flg"
  [VACC_EcasSw3Knee_flg] -> Switch24/3
  Equal2/1 -> Switch24/1
  [VINP_CP2VKneeReqRSide_enum] -> Equal2/1
  Constant22/1 -> Switch25/1
  Bus Selector/16 -> [VINP_CP2VKneeReqRSide_enum]  "<VINP_CP2VKneeReqRSide_enum>"
  OR/1 -> Switch25/2
  [VDMM_DTCECASButWireFailure_flg] -> OR/2
  [VDSC_ECASKneeSideSW_flg] -> OR/1
  [VDMM_DTCECASButWireFailure_flg] -> OR1/2
  OR1/1 -> Switch27/2
  Constant24/1 -> Switch27/1
  [VINP_CP2VKneeReqRSide_enum] -> Equal3/1
  Equal3/1 -> Switch26/1
  [VACC_EcasSw3Knee_flg] -> Switch26/3
  Switch27/1 -> [VACC_ASC2KneeReqRSide_flg]  "VACC_ASC2KneeReqRSide_flg"
  [VDSC_ECASSwitch_flg] -> NOT13/1
  Switch26/1 -> Switch27/3
  NOT13/1 -> Switch26/2
  Constant25/1 -> Equal3/2
  [VDSC_ECASKneeSideSW_flg] -> NOT14/1
  NOT14/1 -> OR1/1
  [VACC_ASC2AutoTracH_enum] -> VACC_ASC2AutoTracH_enum/1
  [VACC_ASC2KneeCtrlMReq_enum] -> VACC_ASC2KneeCtrlMReq_enum/1
  [VACC_ASC2NLvReqFA_enum] -> VACC_ASC2NLvReqFA_enum/1
  [VACC_ASC2NLvReqRA_enum] -> VACC_ASC2NLvReqRA_enum/1
  [VACC_ASC2LvCtrlModeReq_enum] -> VACC_ASC2LvCtrlModeReq_enum/1
  [VACC_ASC2LA1PosCmd_enum] -> VACC_ASC2LA1PosCmd_enum/1
  [VACC_ASC2LA2PosCmd_enum] -> VACC_ASC2LA2PosCmd_enum/1
  [VACC_ASC2DamStiffReqFA_pct] -> VACC_ASC2DamStiffReqFA_pct/1
  [VACC_ASC2DamStiffReqRA_pct] -> VACC_ASC2DamStiffReqRA_pct/1
  [VACC_ASC2DamStiffReqLA_pct] -> VACC_ASC2DamStiffReqLA_pct/1
  [VACC_ASC2KneeReqFA_flg] -> VACC_ASC2KneeReqFA_flg/1
  [VACC_ASC2KneeReqRA_flg] -> VACC_ASC2KneeReqRA_flg/1
  [VACC_ASC2KneeReqLSide_flg] -> VACC_ASC2KneeReqLSide_flg/1
  [VACC_ASC2KneeReqRSide_flg] -> VACC_ASC2KneeReqRSide_flg/1

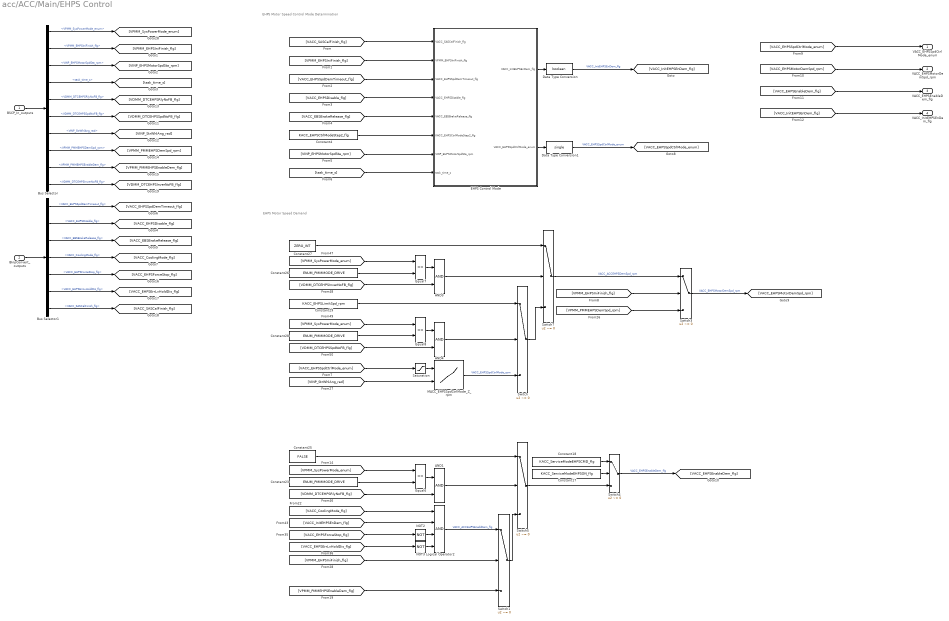
== system acc/ACC/Main/EHPS Control ==
  note: EHPS Motor Speed Demand
  note: EHPS Motor Speed Control Mode Determination
  BSCP_In_outputs : Inport
  BInpConvert_outputs : Inport  Port=2
  AND1 : Logic  AllPortsSameDT=off  OutDataTypeStr=boolean
  AND3 : Logic  AllPortsSameDT=off  OutDataTypeStr=boolean
  AND4 : Logic  AllPortsSameDT=off  OutDataTypeStr=boolean
  Bus Selector : BusSelector  OutputSignals=VPMM_SysPowerMode_enum,VPMM_EHPSIniFinish_flg,VINP_EHPSMotorSpdSta_rpm,task_time_s,VDMM_DTCEHPSRlyNoFB_flg,VDMM_DTCEHPSSpdNoFB_flg,VINP_StrWhlAng_rad,VPMM_PMMEHPSDemSpd_rpm,VPMM_PMMEHPSEnableDem_flg,VDMM_DTCEHPSInverNoFB_flg
  Bus Selector1 : BusSelector  OutputSignals=VACC_EHPSSpdDemTimeout_flg,VACC_EHPSDisable_flg,VACC_EBSBrakeRelease_flg,VACC_CoolingMode_flg,VACC_EHPSForceStop_flg,VACC_EHPSErrLvHoldDis_flg,VACC_SASCalFinish_flg
  Constant17 : Constant  Value=KACC_ServiceModeEHPSON_flg
  Constant18 : Constant  Value=KACC_ServiceModeEHPSCMD_flg
  Constant23 : Constant  Value=ENUM_PMMMODE_DRIVE  SampleTime=-1
  Constant25 : Constant  Value=FALSE
  Constant26 : Constant  Value=ENUM_PMMMODE_DRIVE  SampleTime=-1
  Constant27 : Constant  Value=ZERO_INT
  Constant28 : Constant  Value=ENUM_PMMMODE_DRIVE  SampleTime=-1
  Constant29 : Constant  Value=KACC_EHPSLimitSpd_rpm  SampleTime=-1
  Constant4 : Constant  Value=KACC_EHPSCtrlModeStep2_flg  SampleTime=-1
  Data Type Conversion : DataTypeConversion  OutDataTypeStr=boolean
  Data Type Conversion1 : DataTypeConversion  OutDataTypeStr=single
  EHPS Control Mode : Stateflow chart  TreatAsAtomicUnit=on
  Equal6 : RelationalOperator  Operator===  OutDataTypeStr=boolean  RndMeth=Simplest
  Equal7 : RelationalOperator  Operator===  OutDataTypeStr=boolean  RndMeth=Simplest
  Equal8 : RelationalOperator  Operator===  OutDataTypeStr=boolean  RndMeth=Simplest
  Logical Operator2 : Logic  Inputs=4  AllPortsSameDT=off  OutDataTypeStr=boolean
  MACC_EHPSSpdCtrlMode_Z_rpm : Lookup_n-D  BreakpointsForDimension1=AACC_EHPSSpdCtrlMode_Y_rad  BreakpointsForDimension2=AACC_EHPSSpdCtrlMode_X_enum  Table=MACC_EHPSSpdCtrlMode_Z_rpm  InternalRulePriority=Speed  RndMeth=Simplest  InputSameDT=on
      settings: InputPortMap=u0,u1
  NOT2 : Logic  Operator=NOT  AllPortsSameDT=off  OutDataTypeStr=boolean
  NOT3 : Logic  Operator=NOT  AllPortsSameDT=off  OutDataTypeStr=boolean
  Saturation : Saturate  UpperLimit=4  LowerLimit=1
      settings: AttributesFormatString=|
      | UpperLimit:%<UpperLimit>
      | LowerLimi:%<LowerLimit>
  Switch{,1,3..5,7} (6 alike) : Switch  Criteria=u2 ~= 0
      settings: AttributesFormatString=%<Criteria>
  VACC_EHPSSpdCtrlMode_enum : Outport
  VACC_EHPSMotorDemSpd_rpm : Outport  Port=2
  VACC_EHPSEnableDem_flg : Outport  Port=3
  VACC_InitEHPSEnDem_flg : Outport  Port=4
  wires:
  BSCP_In_outputs/1 -> Bus Selector/1
  BInpConvert_outputs/1 -> Bus Selector1/1
  [VACC_SASCalFinish_flg] -> EHPS Control Mode/1(VACC_SASCalFinish_flg)
  [VPMM_EHPSIniFinish_flg] -> EHPS Control Mode/2(VPMM_EHPSIniFinish_flg)
  [VACC_EHPSSpdDemTimeout_flg] -> EHPS Control Mode/3(VACC_EHPSSpdDemTimeout_flg)
  [VACC_EHPSDisable_flg] -> EHPS Control Mode/4(VACC_EHPSDisable_flg)
  [VACC_EBSBrakeRelease_flg] -> EHPS Control Mode/5(VACC_EBSBrakeRelease_flg)
  [VINP_EHPSMotorSpdSta_rpm] -> EHPS Control Mode/7(VINP_EHPSMotorSpdSta_rpm)
  [task_time_s] -> EHPS Control Mode/8(task_time_s)
  Constant4/1 -> EHPS Control Mode/6(KACC_EHPSCtrlModeStep2_flg)
  EHPS Control Mode/1(VACC_InitEHPSEnDem_flg) -> Data Type Conversion/1
  Data Type Conversion/1 -> [VACC_InitEHPSEnDem_flg]  "VACC_InitEHPSEnDem_flg"
  EHPS Control Mode/2(VACC_EHPSSpdCtrlMode_enum) -> Data Type Conversion1/1
  Data Type Conversion1/1 -> [VACC_EHPSSpdCtrlMode_enum]  "VACC_EHPSSpdCtrlMode_enum"
  [VINP_StrWhlAng_rad] -> MACC_EHPSSpdCtrlMode_Z_rpm/2
  [VPMM_EHPSIniFinish_flg] -> Switch3/2
  AND4/1 -> Switch/2
  Saturation/1 -> MACC_EHPSSpdCtrlMode_Z_rpm/1
  Constant28/1 -> Equal8/2
  [VDMM_DTCEHPSInverNoFB_flg] -> AND3/2
  Equal7/1 -> AND3/1
  [VPMM_PMMEHPSDemSpd_rpm] -> Switch3/3
  AND3/1 -> Switch7/2
  Equal8/1 -> AND4/1
  Constant26/1 -> Equal7/2
  [VDMM_DTCEHPSSpdNoFB_flg] -> AND4/2
  Constant27/1 -> Switch7/1
  Constant29/1 -> Switch/1
  Switch7/1 -> Switch3/1  "VACC_ACCEHPSDemSpd_rpm"
  [VPMM_SysPowerMode_enum] -> Equal7/1
  [VPMM_SysPowerMode_enum] -> Equal8/1
  Switch/1 -> Switch7/3
  MACC_EHPSSpdCtrlMode_Z_rpm/1 -> Switch/3  "VACC_EHPSSpdCtrlMode_rpm"
  [VACC_EHPSSpdCtrlMode_enum] -> Saturation/1
  Switch3/1 -> [VACC_EHPSMotorDemSpd_rpm]  "VACC_EHPSMotorDemSpd_rpm"
  [VDMM_DTCEHPSRlyNoFB_flg] -> AND1/2
  Constant25/1 -> Switch5/1
  Switch1/1 -> Switch5/3
  Switch5/1 -> Switch4/3
  AND1/1 -> Switch5/2
  Constant23/1 -> Equal6/2
  [VPMM_SysPowerMode_enum] -> Equal6/1
  Equal6/1 -> AND1/1
  [VPMM_PMMEHPSEnableDem_flg] -> Switch1/3
  Constant17/1 -> Switch4/2
  Constant18/1 -> Switch4/1
  [VPMM_EHPSIniFinish_flg] -> Switch1/2
  [VACC_InitEHPSEnDem_flg] -> Logical Operator2/2
  NOT2/1 -> Logical Operator2/3
  [VACC_EHPSErrLvHoldDis_flg] -> NOT3/1
  [VACC_EHPSForceStop_flg] -> NOT2/1
  NOT3/1 -> Logical Operator2/4
  Logical Operator2/1 -> Switch1/1  "VACC_ACCEHPSEnablDem_flg"
  [VACC_CoolingMode_flg] -> Logical Operator2/1
  Switch4/1 -> [VACC_EHPSEnableDem_flg]  "VACC_EHPSEnableDem_flg"
  [VACC_EHPSSpdCtrlMode_enum] -> VACC_EHPSSpdCtrlMode_enum/1
  [VACC_EHPSMotorDemSpd_rpm] -> VACC_EHPSMotorDemSpd_rpm/1
  [VACC_EHPSEnableDem_flg] -> VACC_EHPSEnableDem_flg/1
  Bus Selector/1 -> [VPMM_SysPowerMode_enum]  "<VPMM_SysPowerMode_enum>"
  Bus Selector/2 -> [VPMM_EHPSIniFinish_flg]  "<VPMM_EHPSIniFinish_flg>"
  Bus Selector/3 -> [VINP_EHPSMotorSpdSta_rpm]  "<VINP_EHPSMotorSpdSta_rpm>"
  Bus Selector/4 -> [task_time_s]  "<task_time_s>"
  Bus Selector/5 -> [VDMM_DTCEHPSRlyNoFB_flg]  "<VDMM_DTCEHPSRlyNoFB_flg>"
  Bus Selector/6 -> [VDMM_DTCEHPSSpdNoFB_flg]  "<VDMM_DTCEHPSSpdNoFB_flg>"
  Bus Selector/7 -> [VINP_StrWhlAng_rad]  "<VINP_StrWhlAng_rad>"
  Bus Selector/8 -> [VPMM_PMMEHPSDemSpd_rpm]  "<VPMM_PMMEHPSDemSpd_rpm>"
  Bus Selector/9 -> [VPMM_PMMEHPSEnableDem_flg]  "<VPMM_PMMEHPSEnableDem_flg>"
  Bus Selector1/1 -> [VACC_EHPSSpdDemTimeout_flg]  "<VACC_EHPSSpdDemTimeout_flg>"
  Bus Selector1/2 -> [VACC_EHPSDisable_flg]  "<VACC_EHPSDisable_flg>"
  Bus Selector1/3 -> [VACC_EBSBrakeRelease_flg]  "<VACC_EBSBrakeRelease_flg>"
  Bus Selector1/4 -> [VACC_CoolingMode_flg]  "<VACC_CoolingMode_flg>"
  Bus Selector1/5 -> [VACC_EHPSForceStop_flg]  "<VACC_EHPSForceStop_flg>"
  Bus Selector1/6 -> [VACC_EHPSErrLvHoldDis_flg]  "<VACC_EHPSErrLvHoldDis_flg>"
  Bus Selector1/7 -> [VACC_SASCalFinish_flg]  "<VACC_SASCalFinish_flg>"
  Bus Selector/10 -> [VDMM_DTCEHPSInverNoFB_flg]  "<VDMM_DTCEHPSInverNoFB_flg>"
  [VACC_InitEHPSEnDem_flg] -> VACC_InitEHPSEnDem_flg/1

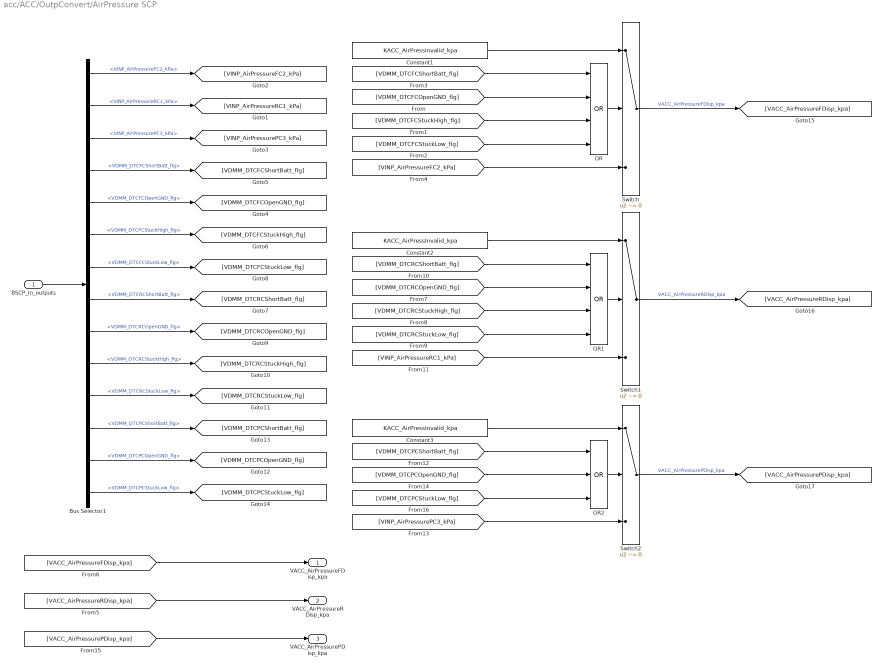
== system acc/ACC/OutpConvert/AirPressure SCP ==
  BSCP_In_outputs : Inport
  Bus Selector1 : BusSelector  OutputSignals=VINP_AirPressureFC2_kPa,VINP_AirPressureRC1_kPa,VINP_AirPressurePC3_kPa,VDMM_DTCFCShortBatt_flg,VDMM_DTCFCOpenGND_flg,VDMM_DTCFCStuckHigh_flg,VDMM_DTCFCStuckLow_flg,VDMM_DTCRCShortBatt_flg,VDMM_DTCRCOpenGND_flg,VDMM_DTCRCStuckHigh_flg,VDMM_DTCRCStuckLow_flg,VDMM_DTCPCShortBatt_flg,VDMM_DTCPCOpenGND_flg,VDMM_DTCPCStuckLow_flg
  Constant1 : Constant  Value=KACC_AirPressInvalid_kpa
  Constant2 : Constant  Value=KACC_AirPressInvalid_kpa
  Constant3 : Constant  Value=KACC_AirPressInvalid_kpa
  OR : Logic  Operator=OR  Inputs=4  AllPortsSameDT=off  OutDataTypeStr=boolean
  OR1 : Logic  Operator=OR  Inputs=4  AllPortsSameDT=off  OutDataTypeStr=boolean
  OR2 : Logic  Operator=OR  Inputs=3  AllPortsSameDT=off  OutDataTypeStr=boolean
  Switch : Switch  Criteria=u2 ~= 0
      settings: AttributesFormatString=%<Criteria>
  Switch1 : Switch  Criteria=u2 ~= 0
      settings: AttributesFormatString=%<Criteria>
  Switch2 : Switch  Criteria=u2 ~= 0
      settings: AttributesFormatString=%<Criteria>
  VACC_AirPressureFDisp_kpa : Outport
  VACC_AirPressureRDisp_kpa : Outport  Port=2
  VACC_AirPressurePDisp_kpa : Outport  Port=3
  wires:
  [VACC_AirPressureRDisp_kpa] -> VACC_AirPressureRDisp_kpa/1
  [VACC_AirPressureFDisp_kpa] -> VACC_AirPressureFDisp_kpa/1
  Bus Selector1/3 -> [VINP_AirPressurePC3_kPa]  "<VINP_AirPressurePC3_kPa>"
  Bus Selector1/2 -> [VINP_AirPressureRC1_kPa]  "<VINP_AirPressureRC1_kPa>"
  Bus Selector1/1 -> [VINP_AirPressureFC2_kPa]  "<VINP_AirPressureFC2_kPa>"
  BSCP_In_outputs/1 -> Bus Selector1/1
  Bus Selector1/4 -> [VDMM_DTCFCShortBatt_flg]  "<VDMM_DTCFCShortBatt_flg>"
  Bus Selector1/5 -> [VDMM_DTCFCOpenGND_flg]  "<VDMM_DTCFCOpenGND_flg>"
  Bus Selector1/6 -> [VDMM_DTCFCStuckHigh_flg]  "<VDMM_DTCFCStuckHigh_flg>"
  Bus Selector1/7 -> [VDMM_DTCFCStuckLow_flg]  "<VDMM_DTCFCStuckLow_flg>"
  Bus Selector1/8 -> [VDMM_DTCRCShortBatt_flg]  "<VDMM_DTCRCShortBatt_flg>"
  Bus Selector1/9 -> [VDMM_DTCRCOpenGND_flg]  "<VDMM_DTCRCOpenGND_flg>"
  Bus Selector1/10 -> [VDMM_DTCRCStuckHigh_flg]  "<VDMM_DTCRCStuckHigh_flg>"
  Bus Selector1/11 -> [VDMM_DTCRCStuckLow_flg]  "<VDMM_DTCRCStuckLow_flg>"
  Bus Selector1/12 -> [VDMM_DTCPCShortBatt_flg]  "<VDMM_DTCPCShortBatt_flg>"
  Bus Selector1/13 -> [VDMM_DTCPCOpenGND_flg]  "<VDMM_DTCPCOpenGND_flg>"
  Bus Selector1/14 -> [VDMM_DTCPCStuckLow_flg]  "<VDMM_DTCPCStuckLow_flg>"
  [VDMM_DTCFCShortBatt_flg] -> OR/1
  [VDMM_DTCFCOpenGND_flg] -> OR/2
  [VDMM_DTCFCStuckHigh_flg] -> OR/3
  [VDMM_DTCFCStuckLow_flg] -> OR/4
  OR/1 -> Switch/2
  [VINP_AirPressureFC2_kPa] -> Switch/3
  Constant1/1 -> Switch/1
  Switch/1 -> [VACC_AirPressureFDisp_kpa]  "VACC_AirPressureFDisp_kpa"
  Switch1/1 -> [VACC_AirPressureRDisp_kpa]  "VACC_AirPressureRDisp_kpa"
  Constant2/1 -> Switch1/1
  [VINP_AirPressureRC1_kPa] -> Switch1/3
  OR1/1 -> Switch1/2
  [VDMM_DTCRCShortBatt_flg] -> OR1/1
  [VDMM_DTCRCOpenGND_flg] -> OR1/2
  [VDMM_DTCRCStuckHigh_flg] -> OR1/3
  [VDMM_DTCRCStuckLow_flg] -> OR1/4
  OR2/1 -> Switch2/2
  Constant3/1 -> Switch2/1
  Switch2/1 -> [VACC_AirPressurePDisp_kpa]  "VACC_AirPressurePDisp_kpa"
  [VINP_AirPressurePC3_kPa] -> Switch2/3
  [VDMM_DTCPCShortBatt_flg] -> OR2/1
  [VDMM_DTCPCOpenGND_flg] -> OR2/2
  [VDMM_DTCPCStuckLow_flg] -> OR2/3
  [VACC_AirPressurePDisp_kpa] -> VACC_AirPressurePDisp_kpa/1

== system acc/ACC/OutpConvert/EAC Pressure Indication ==
  BSCP_In_outputs : Inport
  Bus Selector : BusSelector  OutputSignals=VINP_AirPressureRC1_kPa,VINP_AirPressureFC2_kPa,VINP_AirPressurePC3_kPa
  Constant : Constant  Value=KACC_CACPresWarn_ovrdflg_flg
  Constant1 : Constant  Value=KACC_CACPresWarn_ovrdval_flg
  Constant2 : Constant  Value=KACC_CACPresWarn_kPa
  Constant3 : Constant  Value=KACC_CACPresWarn_kPa
  Constant4 : Constant  Value=KACC_CACPresWarn_kPa
  Logical Operator2 : Logic  Operator=OR  Inputs=3  AllPortsSameDT=off  OutDataTypeStr=boolean
  NOT : Logic  Operator=NOT  AllPortsSameDT=off  OutDataTypeStr=boolean
  Relational Operator1 : RelationalOperator  Operator=<=  OutDataTypeStr=boolean  RndMeth=Simplest
  Relational Operator10 : RelationalOperator  Operator=<=  OutDataTypeStr=boolean  RndMeth=Simplest
  Relational Operator9 : RelationalOperator  Operator=<=  OutDataTypeStr=boolean  RndMeth=Simplest
  Switch1 : Switch  Criteria=u2 ~= 0
      settings: AttributesFormatString=%<Criteria>
  VACC_CACPresWarn_flg : Outport  VectorParamsAs1DForOutWhenUnconnected=off
  VACC_CACPresReady_flg : Outport  Port=2  VectorParamsAs1DForOutWhenUnconnected=off
  wires:
  Relational Operator1/1 -> Logical Operator2/3
  [VINP_AirPressurePC3_kPa] -> Relational Operator1/1
  Switch1/1 -> [VACC_CACPresWarn_flg], NOT/1  "VACC_CACPresWarn_flg"
  Logical Operator2/1 -> Switch1/3
  Constant/1 -> Switch1/2
  Relational Operator10/1 -> Logical Operator2/2
  Constant1/1 -> Switch1/1
  Relational Operator9/1 -> Logical Operator2/1
  [VINP_AirPressureFC2_kPa] -> Relational Operator9/1
  [VINP_AirPressureRC1_kPa] -> Relational Operator10/1
  BSCP_In_outputs/1 -> Bus Selector/1
  Bus Selector/2 -> [VINP_AirPressureFC2_kPa]  "<VINP_AirPressureFC2_kPa>"
  Bus Selector/1 -> [VINP_AirPressureRC1_kPa]  "<VINP_AirPressureRC1_kPa>"
  Bus Selector/3 -> [VINP_AirPressurePC3_kPa]  "<VINP_AirPressurePC3_kPa>"
  Constant4/1 -> Relational Operator1/2
  Constant3/1 -> Relational Operator10/2
  Constant2/1 -> Relational Operator9/2
  NOT/1 -> [VACC_CACPresReady_flg]  "VACC_CACPresReady_flg"
  [VACC_CACPresWarn_flg] -> VACC_CACPresWarn_flg/1
  [VACC_CACPresReady_flg] -> VACC_CACPresReady_flg/1

== system acc/ACC/OutpConvert/EAC Temperature Over High Detection ==
  BSCP_In_outputs : Inport
  Bus Selector : BusSelector  OutputSignals=task_time_s,VINP_CACTemp_C
  Constant1 : Constant  Value=KACC_CACOverTempDelayTime_s
  Constant10 : Constant  Value=KACC_DTCACCReset_flg
  Constant2 : Constant  Value=KACC_CACTempWarn_C
  Constant3 : Constant  Value=KACC_CACOverTempRcv_s
  Constant4 : Constant  Value=ONE_INT
  Constant5 : Constant  Value=KACC_CACTempRev_C
  DTC_Couter : hcu_lib/Basic_Blocks/DTC_Couter
      settings: SourceProductName=HCU Relative Block Library
  Fault : hcu_lib/Basic_Blocks/Fault  SystemSampleTime=-1  VariantActivationTime=update diagram  Latency=0  AutoFrameSizeCalculation=off
      settings: SourceProductName=HCU Relative Block Library
  OR : Logic  Operator=OR  AllPortsSameDT=off  OutDataTypeStr=boolean
  Recover : hcu_lib/Basic_Blocks/Recover  SystemSampleTime=-1  VariantActivationTime=update diagram  Latency=0  AutoFrameSizeCalculation=off
      settings: SourceProductName=HCU Relative Block Library
  Relational Operator2 : RelationalOperator  Operator=<=  OutDataTypeStr=boolean  RndMeth=Simplest
  Relational Operator4 : RelationalOperator  OutDataTypeStr=boolean  RndMeth=Simplest
  Terminator1 : Terminator
  VACC_CACTempOverHigh_flg : Outport
  wires:
  Constant10/1 -> OR/2
  [VINP_CACTemp_C] -> Relational Operator2/1
  Fault/1 -> DTC_Couter/1
  OR/1 -> DTC_Couter/2
  Recover/1 -> OR/1
  [VINP_CACTemp_C] -> Relational Operator4/1
  Relational Operator4/1 -> Fault/2
  [task_time_s] -> Recover/1
  Constant3/1 -> Recover/3
  DTC_Couter/2 -> Terminator1/1
  Relational Operator2/1 -> Recover/2
  Constant4/1 -> DTC_Couter/3
  [task_time_s] -> Fault/1
  Constant1/1 -> Fault/3
  BSCP_In_outputs/1 -> Bus Selector/1
  Constant2/1 -> Relational Operator4/2
  Constant5/1 -> Relational Operator2/2
  Bus Selector/1 -> [task_time_s]  "<task_time_s>"
  Bus Selector/2 -> [VINP_CACTemp_C]  "<VINP_CACTemp_C>"
  DTC_Couter/1 -> [VACC_CACTempOverHigh_flg]  "VACC_CACTempOverHigh_flg"
  [VACC_CACTempOverHigh_flg] -> VACC_CACTempOverHigh_flg/1
